simulink model "sim6"  (R2020a)
settings: Solver=VariableStepAuto  StartTime=0.0  StopTime=10.0  RelTol=1e-3
undefined symbols (not defined in the file): A, B, C1, C2
libraries: eeLuenbergerObserver x4
settings Model: Creator=me-clab2  LastModifiedBy=me-clab2

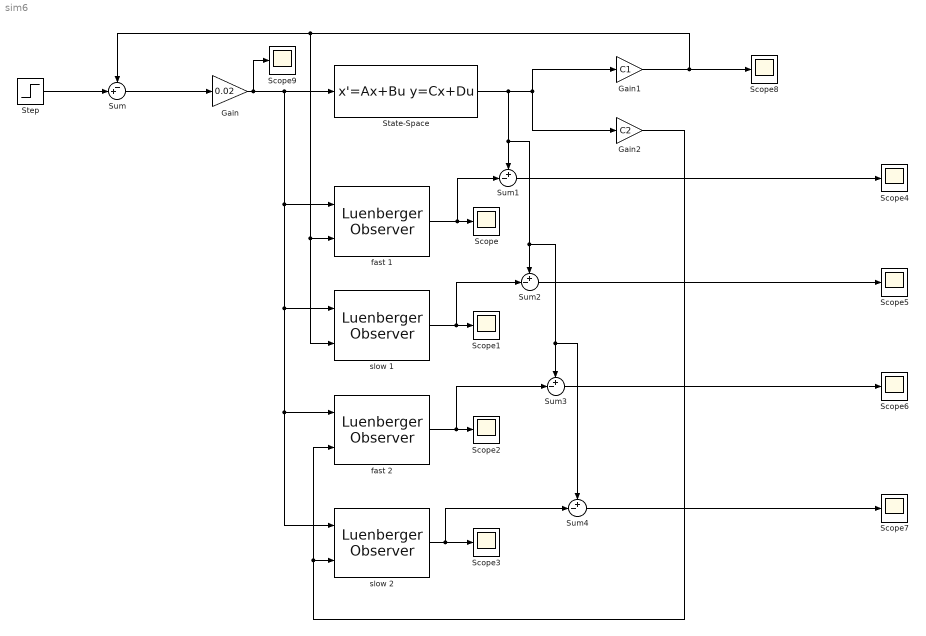
== system sim6 ==
  Gain : Gain  Gain=0.02
  Gain1 : Gain  Gain=C1
  Gain2 : Gain  Gain=C2
  Scope{,1..9} (10 alike) : Scope
  State-Space : StateSpace  A=A  B=B  C=eye(4)  D=[0;0;0;0]  InitialCondition=[30;0;0;0]
  Step : Step  Time=0  After=0  SampleTime=0
  Sum : Sum  Inputs=-+|
  Sum{1..4} (4 alike) : Sum  Inputs=+-|
  fast 1 : eeLuenbergerObserver/Luenberger Observer  StateSpaceType=Continuous-time  Ad=1  Bd=1  Cd=1  Dd=1  A=A  B=B  C=C1  D=0  ObserverDesign=Desired eigenvalues  Ld=1  DesiredEigenvalues=[-9.96 -9.97 -9.98 -9.99]  x0=[0 0 0 0]  Tsd=0.1  Ts=0.001
      settings: SourceProductBaseCode=PS
  fast 2 : eeLuenbergerObserver/Luenberger Observer  StateSpaceType=Continuous-time  Ad=1  Bd=1  Cd=1  Dd=1  A=A  B=B  C=C2  D=[0;0]  ObserverDesign=Desired eigenvalues  Ld=1  DesiredEigenvalues=[-9.96 -9.97 -9.98 -9.99]  x0=[0 0 0 0]  Tsd=0.1  Ts=0.001
      settings: SourceProductBaseCode=PS
  slow 1 : eeLuenbergerObserver/Luenberger Observer  StateSpaceType=Continuous-time  Ad=1  Bd=1  Cd=1  Dd=1  A=A  B=B  C=C1  D=0  ObserverDesign=Desired eigenvalues  Ld=1  DesiredEigenvalues=[-1.01 -1.02 -1.03 -1.04]  x0=[0 0 0 0]  Tsd=0.1  Ts=0.001
      settings: SourceProductBaseCode=PS
  slow 2 : eeLuenbergerObserver/Luenberger Observer  StateSpaceType=Continuous-time  Ad=1  Bd=1  Cd=1  Dd=1  A=A  B=B  C=C2  D=[0;0]  ObserverDesign=Desired eigenvalues  Ld=1  DesiredEigenvalues=[-1.01 -1.02 -1.03 -1.04]  x0=[0 0 0 0]  Tsd=0.1  Ts=0.001
      settings: SourceProductBaseCode=PS
  wires:
  Sum/1 -> Gain/1
  Gain/1 -> Scope9/1, slow 2/1, fast 2/1, slow 1/1, fast 1/1, State-Space/1
  fast 1/1 -> Sum1/2, Scope/1
  fast 2/1 -> Sum3/2, Scope2/1
  slow 2/1 -> Sum4/2, Scope3/1
  Gain2/1 -> fast 2/2, slow 2/2
  Gain1/1 -> Scope8/1, slow 1/2, fast 1/2, Sum/1
  Sum1/1 -> Scope4/1
  slow 1/1 -> Sum2/2, Scope1/1
  State-Space/1 -> Sum4/1, Sum3/1, Sum2/1, Sum1/1, Gain2/1, Gain1/1
  Sum2/1 -> Scope5/1
  Sum3/1 -> Scope6/1
  Sum4/1 -> Scope7/1
  Step/1 -> Sum/2
